simulink library "vlbi_lib"  (Simulink 7.3)
settings: Solver=ode45  SolverMode=SingleTasking  StartTime=0.0  StopTime=10.0  RelTol=1e-3
libraries: xbsIndex_r4 x437, xbsReplacements_r4 x26, simulink x3, xps_library x2
(part 1 of 2)
settings Model: Creator=rprimian  LastModifiedBy=rprimian

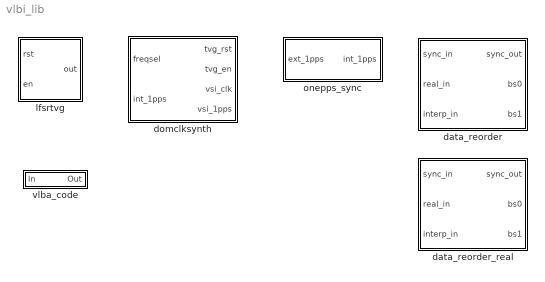
== system vlbi_lib ==
  data_reorder : Subsystem  mask{sample_width=2, vsi_clock=32 MHz}
      mask prompts: sample_width "Channel sample width:"; vsi_clock "VSI output clock rate:"
      mask init:
      | myname = gcb;
      | 
      | if (strcmp(vsi_clock, '32 MHz'))
      |     set_param([gcb, '/sync2rd'], 'latency', '4');
      |     set_param([gcb, '/rdaddrcount'], 'n_bits', '4');
      |     set_param([gcb, '/rdaddrtopslice'], 'nbits', '3');
      |     set_param([gcb, '/wraddrcount'], 'n_bits', '4');
      |     set_param([gcb, '/sync2align'], 'latency', '7');
      |     set_param([gcb, '/aligncount'], 'n_bits', '3');
      |     set_param([gcb, '/alignconst'], 'n_bits', '3');
      |     set_param([gcb, '/reorder_bram'], 'depth', '32');
      | elseif (strcmp(vsi_clock, '64 MHz'))
      |     set_param([gcb, '/sync2rd'], 'latency', '2');
      |     set_param([gcb, '/rdaddrcount'], 'n_bits', '3');
      |     set_param([gcb, '/rdaddrtopslice'], 'nbits', '2');
      |     set_param([gcb, '/wraddrcount'], 'n_bits', '3');
      |     set_param([gcb, '/sync2align'], 'latency', '5');
      |     set_param([gcb, '/aligncount'], 'n_bits', '2');
      |     set_param([gcb, '/alignconst'], 'n_bits', '2');
      |     set_param([gcb, '/reorder_bram'], 'depth', '16');
      | end
      mask StyleString: edit,popup(32 MHz|64 MHz)
  data_reorder_real : Subsystem  mask{sample_width=8, vsi_clock=32 MHz}
      mask prompts: sample_width "Channel sample width:"; vsi_clock "VSI output clock rate:"
      mask init:
      | myname = gcb;
      | 
      | if (strcmp(vsi_clock, '32 MHz'))
      |     set_param([gcb, '/restream'], 'clock_rate', '32');
      |     set_param([gcb, '/slc_wrmask'], 'bit1', '-1');
      | else
      |     set_param([gcb, '/restream'], 'clock_rate', '64');
      |     set_param([gcb, '/slc_wrmask'], 'bit1', '0');
      | end
      mask StyleString: edit,popup(32 MHz|64 MHz)
  domclksynth : Subsystem
  lfsrtvg : Subsystem
  onepps_sync : Subsystem
  vlba_code : Subsystem  mask{bitwidth=18}
      mask prompts: bitwidth "Rounding bitwidth:"
      mask Display: fprintf('z^-4')

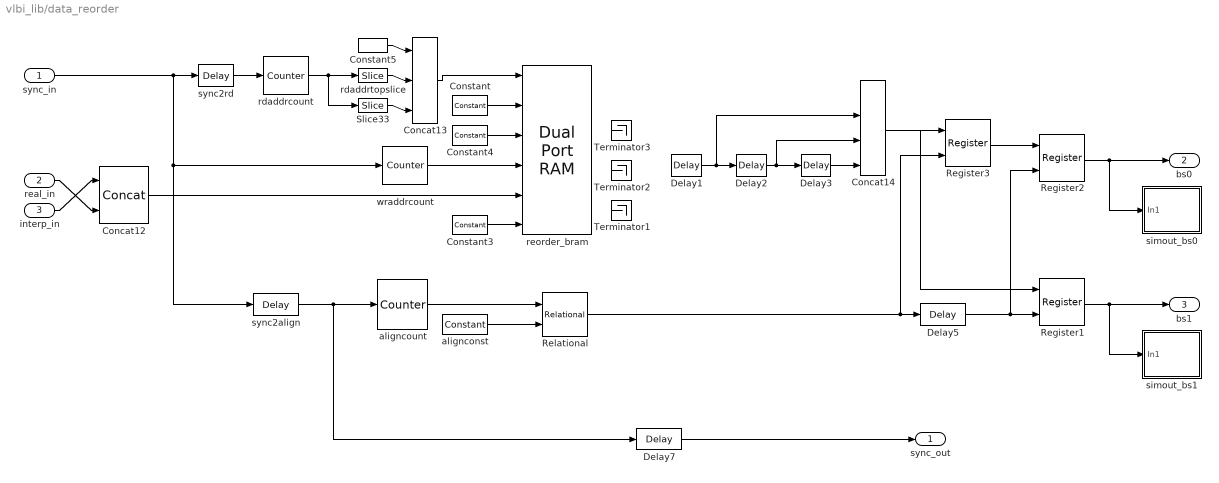
== system vlbi_lib/data_reorder ==
  sync_in : Inport  OutDataType=sfix(16)  OutScaling=2^0
  real_in : Inport  Port=2  OutDataType=sfix(16)  OutScaling=2^0
  interp_in : Inport  Port=3  OutDataType=sfix(16)  OutScaling=2^0
  Concat12 : xbsIndex_r4/Concat  num_inputs=2  dbl_ovrd=off  block_type=concat
      settings: block_version=11.3
  Concat13 : xbsIndex_r4/Concat  num_inputs=3  dbl_ovrd=off  block_type=concat
      settings: block_version=11.3
  Concat14 : xbsIndex_r4/Concat  num_inputs=4  dbl_ovrd=off  block_type=concat
      settings: block_version=11.3
  Constant : xbsIndex_r4/Constant  arith_type=Unsigned  const=0  n_bits=sample_width * 4  bin_pt=0  explicit_period=on  period=1  equ=P=C  opselect=C  inp2=PCIN>>17  opr=+  inp1=P  carry=CIN  dbl_ovrd=off  block_type=constant
      settings: block_version=11.3
  Constant3 : xbsIndex_r4/Constant  arith_type=Boolean  const=1  n_bits=1  bin_pt=0  explicit_period=on  period=1  equ=P=C  opselect=C  inp2=PCIN>>17  opr=+  inp1=P  carry=CIN  dbl_ovrd=off  block_type=constant
      settings: block_version=11.3
  Constant4 : xbsIndex_r4/Constant  arith_type=Boolean  const=0  n_bits=1024  bin_pt=0  explicit_period=on  period=1  equ=P=C  opselect=C  inp2=PCIN>>17  opr=+  inp1=P  carry=CIN  dbl_ovrd=off  block_type=constant
      settings: block_version=11.3
  Constant5 : xbsIndex_r4/Constant  arith_type=Unsigned  const=0  n_bits=1  bin_pt=0  explicit_period=on  period=1  equ=P=C  opselect=C  inp2=PCIN>>17  opr=+  inp1=P  carry=CIN  dbl_ovrd=off  block_type=constant
      settings: block_version=11.3
  Delay{1..3,7} (4 alike) : xbsIndex_r4/Delay  en=off  latency=1  dbl_ovrd=off  reg_retiming=off  block_type=delay
      settings: xl_area=[0, 0, 0, 0, 0, 0, 0]  block_version=11.3
  Delay5 : xbsIndex_r4/Delay  en=off  latency=4  dbl_ovrd=off  reg_retiming=off  block_type=delay
      settings: xl_area=[0, 0, 0, 0, 0, 0, 0]  block_version=11.3
  Register1 : xbsIndex_r4/Register  init=0  rst=off  en=on  dbl_ovrd=off  block_type=register
      settings: xl_area=[0, 0, 0, 0, 0, 0, 0]  block_version=11.3
  Register2 : xbsIndex_r4/Register  init=0  rst=off  en=on  dbl_ovrd=off  block_type=register
      settings: xl_area=[0, 0, 0, 0, 0, 0, 0]  block_version=11.3
  Register3 : xbsIndex_r4/Register  init=0  rst=off  en=on  dbl_ovrd=off  block_type=register
      settings: xl_area=[0, 0, 0, 0, 0, 0, 0]  block_version=11.3
  Relational : xbsIndex_r4/Relational  mode=a=b  en=off  latency=1  dbl_ovrd=off  block_type=relational
      settings: xl_area=[0, 0, 0, 0, 0, 0, 0]  block_version=11.3
  Slice33 : xbsIndex_r4/Slice  nbits=1  boolean_output=off  mode=Upper Bit Location + Width  bit1=0  base1=MSB of Input  bit0=0  base0=LSB of Input  dbl_ovrd=off  block_type=slice
      settings: block_version=11.3
  Terminator1 : Terminator
  Terminator2 : Terminator
  Terminator3 : Terminator
  alignconst : xbsIndex_r4/Constant  arith_type=Unsigned  const=0  n_bits=3  bin_pt=0  explicit_period=on  period=1  equ=P=C  opselect=C  inp2=PCIN>>17  opr=+  inp1=P  carry=CIN  dbl_ovrd=off  block_type=constant
      settings: block_version=11.3
  aligncount : xbsIndex_r4/Counter  cnt_type=Free Running  cnt_to=Inf  operation=Up  start_count=0  cnt_by_val=1  arith_type=Unsigned  n_bits=3  bin_pt=0  load_pin=off  rst=on  en=off  explicit_period=off  period=1  dbl_ovrd=off  use_behavioral_HDL=off  implementation=Fabric  use_rpm=on  block_type=counter
      settings: xl_area=[0, 0, 0, 0, 0, 0, 0]  block_version=11.3
  rdaddrcount : xbsIndex_r4/Counter  cnt_type=Free Running  cnt_to=Inf  operation=Up  start_count=0  cnt_by_val=1  arith_type=Unsigned  n_bits=4  bin_pt=0  load_pin=off  rst=on  en=off  explicit_period=off  period=1  dbl_ovrd=off  use_behavioral_HDL=off  implementation=Fabric  use_rpm=on  block_type=counter
      settings: xl_area=[0, 0, 0, 0, 0, 0, 0]  block_version=11.3
  rdaddrtopslice : xbsIndex_r4/Slice  nbits=3  boolean_output=off  mode=Lower Bit Location + Width  bit1=0  base1=MSB of Input  bit0=0  base0=LSB of Input  dbl_ovrd=off  block_type=slice
      settings: block_version=11.3
  reorder_bram : xbsIndex_r4/Dual Port RAM  depth=32  initVector=zeros(32)  distributed_mem=Block RAM  init_a=0  init_b=0  rst_a=off  rst_b=off  en_a=off  en_b=off  latency=1  write_mode_A=Read After Write  write_mode_B=Read After Write  dbl_ovrd=off  optimize=Area  use_rpm=off  block_type=dpram
      settings: xl_area=[0, 0, 0, 0, 0, 0, 0]  block_version=11.3
  simout_bs0 : Subsystem  mask{sample_width=sample_width}
      mask prompts: sample_width "Sample width"
  simout_bs1 : Subsystem  mask{sample_width=sample_width}
      mask prompts: sample_width "Sample width"
  sync2align : xbsIndex_r4/Delay  en=off  latency=7  dbl_ovrd=off  reg_retiming=off  block_type=delay
      settings: xl_area=[0, 0, 0, 0, 0, 0, 0]  block_version=11.3
  sync2rd : xbsIndex_r4/Delay  en=off  latency=4  dbl_ovrd=off  reg_retiming=off  block_type=delay
      settings: xl_area=[0, 0, 0, 0, 0, 0, 0]  block_version=11.3
  wraddrcount : xbsIndex_r4/Counter  cnt_type=Free Running  cnt_to=Inf  operation=Up  start_count=0  cnt_by_val=1  arith_type=Unsigned  n_bits=4  bin_pt=0  load_pin=off  rst=on  en=off  explicit_period=off  period=1  dbl_ovrd=off  use_behavioral_HDL=off  implementation=Fabric  use_rpm=on  block_type=counter
      settings: xl_area=[0, 0, 0, 0, 0, 0, 0]  block_version=11.3
  sync_out : Outport  OutDataType=sfix(16)  OutScaling=2^0
  bs0 : Outport  Port=2  OutDataType=sfix(16)  OutScaling=2^0
  bs1 : Outport  Port=3  OutDataType=sfix(16)  OutScaling=2^0
  wires:
  ? -> Terminator3/1
  Concat12/1 -> reorder_bram/5
  ? -> Terminator1/1
  Constant/1 -> reorder_bram/2
  Constant4/1 -> reorder_bram/3
  rdaddrcount/1 -> rdaddrtopslice/1, Slice33/1
  Constant5/1 -> Concat13/1
  rdaddrtopslice/1 -> Concat13/2
  Slice33/1 -> Concat13/3
  Concat13/1 -> reorder_bram/1
  wraddrcount/1 -> reorder_bram/4
  Constant3/1 -> reorder_bram/6
  Concat14/1 -> Register1/1, Register3/1
  aligncount/1 -> Relational/1
  alignconst/1 -> Relational/2
  Register2/1 -> bs0/1, simout_bs0/1(In1)
  Relational/1 -> Delay5/1, Register3/2
  Register1/1 -> bs1/1, simout_bs1/1(In1)
  Delay5/1 -> Register1/2, Register2/2
  ? -> Terminator2/1
  Register3/1 -> Register2/1
  sync_in/1 -> sync2rd/1, wraddrcount/1, sync2align/1
  sync2rd/1 -> rdaddrcount/1
  real_in/1 -> Concat12/2
  interp_in/1 -> Concat12/1
  sync2align/1 -> aligncount/1, Delay7/1
  Delay7/1 -> sync_out/1
  ? -> Delay1/1, Concat14/1
  Delay2/1 -> Delay3/1, Concat14/3
  Delay1/1 -> Delay2/1, Concat14/2
  Delay3/1 -> Concat14/4

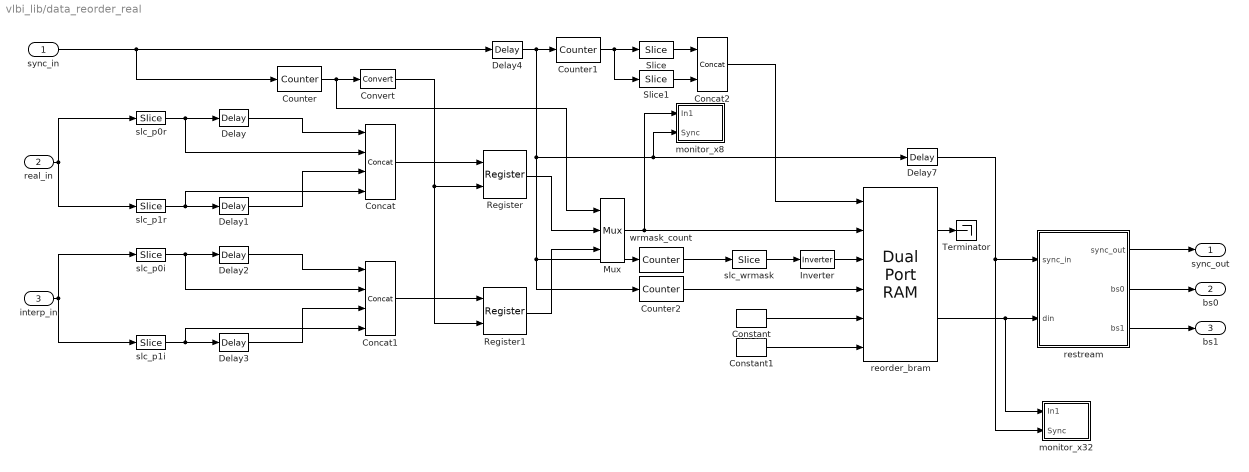
== system vlbi_lib/data_reorder_real ==
  sync_in : Inport  OutDataType=sfix(16)  OutScaling=2^0
  real_in : Inport  Port=2  OutDataType=sfix(16)  OutScaling=2^0
  interp_in : Inport  Port=3  OutDataType=sfix(16)  OutScaling=2^0
  Concat : xbsIndex_r4/Concat  num_inputs=4  dbl_ovrd=off  block_type=concat
      settings: block_version=11.3
  Concat1 : xbsIndex_r4/Concat  num_inputs=4  dbl_ovrd=off  block_type=concat
      settings: block_version=11.3
  Concat2 : xbsIndex_r4/Concat  num_inputs=2  dbl_ovrd=off  block_type=concat
      settings: block_version=11.3
  Constant : xbsIndex_r4/Constant  arith_type=Unsigned  const=0  n_bits=32*sample_width  bin_pt=0  explicit_period=on  period=1  equ=P=C  opselect=C  inp2=PCIN>>17  opr=+  inp1=P  carry=CIN  dbl_ovrd=off  block_type=constant
      settings: block_version=11.3
  Constant1 : xbsIndex_r4/Constant  arith_type=Boolean  const=0  n_bits=8*sample_width  bin_pt=0  explicit_period=on  period=1  equ=P=C  opselect=C  inp2=PCIN>>17  opr=+  inp1=P  carry=CIN  dbl_ovrd=off  block_type=constant
      settings: block_version=11.3
  Convert : xbsIndex_r4/Convert  arith_type=Boolean  n_bits=8  bin_pt=6  quantization=Truncate  overflow=Wrap  latency=0  dbl_ovrd=off  pipeline=off  block_type=convert
      settings: xl_area=[0, 0, 0, 0, 0, 0, 0]  block_version=11.3
  Counter : xbsIndex_r4/Counter  cnt_type=Free Running  cnt_to=Inf  operation=Up  start_count=0  cnt_by_val=1  arith_type=Unsigned  n_bits=1  bin_pt=0  load_pin=off  rst=on  en=off  explicit_period=off  period=1  dbl_ovrd=off  use_behavioral_HDL=off  implementation=Fabric  use_rpm=on  block_type=counter
      settings: xl_area=[0, 0, 0, 0, 0, 0, 0]  block_version=11.3
  Counter1 : xbsIndex_r4/Counter  cnt_type=Free Running  cnt_to=Inf  operation=Up  start_count=0  cnt_by_val=1  arith_type=Unsigned  n_bits=3  bin_pt=0  load_pin=off  rst=on  en=off  explicit_period=off  period=1  dbl_ovrd=off  use_behavioral_HDL=off  implementation=Fabric  use_rpm=on  block_type=counter
      settings: xl_area=[0, 0, 0, 0, 0, 0, 0]  block_version=11.3
  Counter2 : xbsIndex_r4/Counter  cnt_type=Free Running  cnt_to=Inf  operation=Up  start_count=0  cnt_by_val=1  arith_type=Unsigned  n_bits=1  bin_pt=0  load_pin=off  rst=on  en=off  explicit_period=off  period=1  dbl_ovrd=off  use_behavioral_HDL=off  implementation=Fabric  use_rpm=on  block_type=counter
      settings: xl_area=[0, 0, 0, 0, 0, 0, 0]  block_version=11.3
  Delay{,1..3} (4 alike) : xbsIndex_r4/Delay  en=off  latency=1  dbl_ovrd=off  reg_retiming=off  block_type=delay
      settings: xl_area=[0, 0, 0, 0, 0, 0, 0]  block_version=11.3
  Delay4 : xbsIndex_r4/Delay  en=off  latency=3  dbl_ovrd=off  reg_retiming=off  block_type=delay
      settings: xl_area=[0, 0, 0, 0, 0, 0, 0]  block_version=11.3
  Delay7 : xbsIndex_r4/Delay  en=off  latency=11  dbl_ovrd=off  reg_retiming=off  block_type=delay
      settings: xl_area=[0, 0, 0, 0, 0, 0, 0]  block_version=11.3
  Inverter : xbsIndex_r4/Inverter  en=off  latency=0  dbl_ovrd=off  block_type=inv
      settings: xl_area=[0, 0, 0, 0, 0, 0, 0]  block_version=11.3
  Mux : xbsIndex_r4/Mux  inputs=2  en=off  latency=1  precision=Full  arith_type="Signed  (2's comp)"  n_bits=8  bin_pt=2  quantization=Truncate  overflow=Wrap  dbl_ovrd=off  block_type=mux
      settings: xl_area=[0, 0, 0, 0, 0, 0, 0]  block_version=11.3
  Register : xbsIndex_r4/Register  init=0  rst=off  en=on  dbl_ovrd=off  block_type=register
      settings: xl_area=[0, 0, 0, 0, 0, 0, 0]  block_version=11.3
  Register1 : xbsIndex_r4/Register  init=0  rst=off  en=on  dbl_ovrd=off  block_type=register
      settings: xl_area=[0, 0, 0, 0, 0, 0, 0]  block_version=11.3
  Slice : xbsIndex_r4/Slice  nbits=1  boolean_output=off  mode=Lower Bit Location + Width  bit1=0  base1=MSB of Input  bit0=0  base0=LSB of Input  dbl_ovrd=off  block_type=slice
      settings: block_version=11.3
  Slice1 : xbsIndex_r4/Slice  nbits=2  boolean_output=off  mode=Upper Bit Location + Width  bit1=0  base1=MSB of Input  bit0=0  base0=LSB of Input  dbl_ovrd=off  block_type=slice
      settings: block_version=11.3
  Terminator : Terminator
  monitor_x32 : Subsystem
  monitor_x8 : Subsystem
  reorder_bram : xbsIndex_r4/Dual Port RAM  depth=8  initVector=zeros(2)  distributed_mem=Block RAM  init_a=0  init_b=0  rst_a=off  rst_b=off  en_a=off  en_b=off  latency=3  write_mode_A=Read Before Write  write_mode_B=Read Before Write  dbl_ovrd=off  optimize=Area  use_rpm=off  block_type=dpram
      settings: xl_area=[0, 0, 0, 0, 0, 0, 0]  block_version=11.3
  restream : Subsystem  mask{clock_rate=32}
      mask prompts: clock_rate "Clock rate (MHz)"
  slc_p0i : xbsIndex_r4/Slice  nbits=2*sample_width  boolean_output=off  mode=Upper Bit Location + Width  bit1=0  base1=MSB of Input  bit0=0  base0=LSB of Input  dbl_ovrd=off  block_type=slice
      settings: block_version=11.3
  slc_p0r : xbsIndex_r4/Slice  nbits=2*sample_width  boolean_output=off  mode=Upper Bit Location + Width  bit1=0  base1=MSB of Input  bit0=0  base0=LSB of Input  dbl_ovrd=off  block_type=slice
      settings: block_version=11.3
  slc_p1i : xbsIndex_r4/Slice  nbits=2*sample_width  boolean_output=off  mode=Upper Bit Location + Width  bit1=-2*sample_width  base1=MSB of Input  bit0=0  base0=LSB of Input  dbl_ovrd=off  block_type=slice
      settings: block_version=11.3
  slc_p1r : xbsIndex_r4/Slice  nbits=2*sample_width  boolean_output=off  mode=Upper Bit Location + Width  bit1=-2*sample_width  base1=MSB of Input  bit0=0  base0=LSB of Input  dbl_ovrd=off  block_type=slice
      settings: block_version=11.3
  slc_wrmask : xbsIndex_r4/Slice  nbits=1  boolean_output=on  mode=Upper Bit Location + Width  bit1=-1  base1=MSB of Input  bit0=0  base0=LSB of Input  dbl_ovrd=off  block_type=slice
      settings: block_version=11.3
  wrmask_count : xbsIndex_r4/Counter  cnt_type=Count Limited  cnt_to=31  operation=Up  start_count=0  cnt_by_val=1  arith_type=Unsigned  n_bits=6  bin_pt=0  load_pin=off  rst=on  en=off  explicit_period=off  period=1  dbl_ovrd=off  use_behavioral_HDL=off  implementation=Fabric  use_rpm=on  block_type=counter
      settings: xl_area=[0, 0, 0, 0, 0, 0, 0]  block_version=11.3
  sync_out : Outport  OutDataType=sfix(16)  OutScaling=2^0
  bs0 : Outport  Port=2  OutDataType=sfix(16)  OutScaling=2^0
  bs1 : Outport  Port=3  OutDataType=sfix(16)  OutScaling=2^0
  wires:
  real_in/1 -> slc_p0r/1, slc_p1r/1
  interp_in/1 -> slc_p0i/1, slc_p1i/1
  slc_p0r/1 -> Delay/1, Concat/2
  slc_p1r/1 -> Delay1/1, Concat/4
  slc_p0i/1 -> Delay2/1, Concat1/2
  slc_p1i/1 -> Delay3/1, Concat1/4
  Delay/1 -> Concat/1
  Delay1/1 -> Concat/3
  Delay2/1 -> Concat1/1
  Delay3/1 -> Concat1/3
  Concat/1 -> Register/1
  Concat1/1 -> Register1/1
  sync_in/1 -> Counter/1, Delay4/1
  Counter/1 -> Convert/1, Mux/1
  Convert/1 -> Register/2, Register1/2
  Register/1 -> Mux/2
  Register1/1 -> Mux/3
  Constant/1 -> reorder_bram/5
  Constant1/1 -> reorder_bram/6
  Mux/1 -> monitor_x8/1(In1), reorder_bram/2
  slc_wrmask/1 -> Inverter/1
  Delay4/1 -> Counter1/1, Delay7/1, monitor_x8/2(Sync), Counter2/1, wrmask_count/1
  Counter2/1 -> reorder_bram/4
  reorder_bram/1 -> Terminator/1
  Slice/1 -> Concat2/1
  Slice1/1 -> Concat2/2
  Counter1/1 -> Slice/1, Slice1/1
  Concat2/1 -> reorder_bram/1
  Delay7/1 -> restream/1(sync_in), monitor_x32/2(Sync)
  reorder_bram/2 -> restream/2(din), monitor_x32/1(In1)
  restream/1(sync_out) -> sync_out/1
  restream/2(bs0) -> bs0/1
  restream/3(bs1) -> bs1/1
  wrmask_count/1 -> slc_wrmask/1
  Inverter/1 -> reorder_bram/3

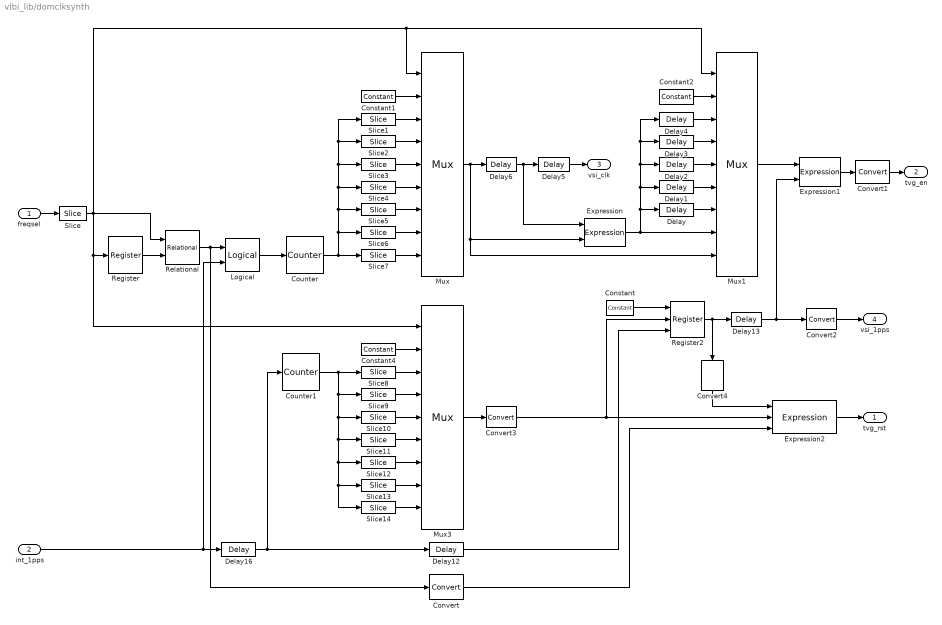
== system vlbi_lib/domclksynth ==
  freqsel : Inport  OutDataType=sfix(16)  OutScaling=2^0
  int_1pps : Inport  Port=2  OutDataType=sfix(16)  OutScaling=2^0
  Constant : xbsIndex_r4/Constant  arith_type=Unsigned  const=1  n_bits=1  bin_pt=0  explicit_period=on  period=1  equ=P=C  opselect=C  inp2=PCIN>>17  opr=+  inp1=P  carry=CIN  dbl_ovrd=off  block_type=constant
      settings: block_version=11.3
  Constant1 : xbsIndex_r4/Constant  arith_type=Unsigned  const=0  n_bits=1  bin_pt=0  explicit_period=on  period=1  equ=P=C  opselect=C  inp2=PCIN>>17  opr=+  inp1=P  carry=CIN  dbl_ovrd=off  block_type=constant
      settings: block_version=11.3
  Constant2 : xbsIndex_r4/Constant  arith_type=Unsigned  const=0  n_bits=1  bin_pt=0  explicit_period=on  period=1  equ=P=C  opselect=C  inp2=PCIN>>17  opr=+  inp1=P  carry=CIN  dbl_ovrd=off  block_type=constant
      settings: block_version=11.3
  Constant4 : xbsIndex_r4/Constant  arith_type=Unsigned  const=0  n_bits=1  bin_pt=0  explicit_period=on  period=1  equ=P=C  opselect=C  inp2=PCIN>>17  opr=+  inp1=P  carry=CIN  dbl_ovrd=off  block_type=constant
      settings: block_version=11.3
  Convert : xbsIndex_r4/Convert  arith_type=Boolean  n_bits=1  bin_pt=0  quantization=Truncate  overflow=Wrap  latency=2  dbl_ovrd=off  pipeline=off  block_type=convert
      settings: xl_area=[0, 0, 0, 0, 0, 0, 0]  block_version=11.3
  Convert{1..4} (4 alike) : xbsIndex_r4/Convert  arith_type=Boolean  n_bits=1  bin_pt=0  quantization=Truncate  overflow=Wrap  latency=0  dbl_ovrd=off  pipeline=off  block_type=convert
      settings: xl_area=[0, 0, 0, 0, 0, 0, 0]  block_version=11.3
  Counter : xbsIndex_r4/Counter  cnt_type=Free Running  cnt_to=Inf  operation=Up  start_count=0  cnt_by_val=1  arith_type=Unsigned  n_bits=8  bin_pt=0  load_pin=off  rst=on  en=off  explicit_period=on  period=1  dbl_ovrd=off  use_behavioral_HDL=off  implementation=Fabric  use_rpm=on  block_type=counter
      settings: xl_area=[0, 0, 0, 0, 0, 0, 0]  block_version=11.3
  Counter1 : xbsIndex_r4/Counter  cnt_type=Free Running  cnt_to=Inf  operation=Up  start_count=0  cnt_by_val=1  arith_type=Unsigned  n_bits=8  bin_pt=0  load_pin=off  rst=on  en=off  explicit_period=on  period=1  dbl_ovrd=off  use_behavioral_HDL=off  implementation=Fabric  use_rpm=on  block_type=counter
      settings: xl_area=[0, 0, 0, 0, 0, 0, 0]  block_version=11.3
  Delay{,5,12,16} (4 alike) : xbsIndex_r4/Delay  en=off  latency=2  dbl_ovrd=off  reg_retiming=off  block_type=delay
      settings: xl_area=[0, 0, 0, 0, 0, 0, 0]  block_version=11.3
  Delay1 : xbsIndex_r4/Delay  en=off  latency=6  dbl_ovrd=off  reg_retiming=off  block_type=delay
      settings: xl_area=[0, 0, 0, 0, 0, 0, 0]  block_version=11.3
  Delay13 : xbsIndex_r4/Delay  en=off  latency=1  dbl_ovrd=off  reg_retiming=off  block_type=delay
      settings: xl_area=[0, 0, 0, 0, 0, 0, 0]  block_version=11.3
  Delay2 : xbsIndex_r4/Delay  en=off  latency=14  dbl_ovrd=off  reg_retiming=off  block_type=delay
      settings: xl_area=[0, 0, 0, 0, 0, 0, 0]  block_version=11.3
  Delay3 : xbsIndex_r4/Delay  en=off  latency=30  dbl_ovrd=off  reg_retiming=off  block_type=delay
      settings: xl_area=[0, 0, 0, 0, 0, 0, 0]  block_version=11.3
  Delay4 : xbsIndex_r4/Delay  en=off  latency=62  dbl_ovrd=off  reg_retiming=off  block_type=delay
      settings: xl_area=[0, 0, 0, 0, 0, 0, 0]  block_version=11.3
  Delay6 : xbsIndex_r4/Delay  en=off  latency=1  dbl_ovrd=off  reg_retiming=off  block_type=delay
      settings: xl_area=[0, 0, 0, 0, 0, 0, 0]  block_version=11.3
  Expression : xbsIndex_r4/Expression  expression=~a & b  align_bp=on  en=off  latency=1  precision=Full  arith_type=Unsigned  n_bits=8  bin_pt=2  dbl_ovrd=off  block_type=expr
      settings: xl_area=[0, 0, 0, 0, 0, 0, 0]  block_version=11.3
  Expression1 : xbsIndex_r4/Expression  expression=a & ~b  align_bp=on  en=off  latency=1  precision=Full  arith_type=Unsigned  n_bits=8  bin_pt=2  dbl_ovrd=off  block_type=expr
      settings: xl_area=[0, 0, 0, 0, 0, 0, 0]  block_version=11.3
  Expression2 : xbsIndex_r4/Expression  expression=(a & b) | c  align_bp=on  en=off  latency=1  precision=Full  arith_type=Unsigned  n_bits=8  bin_pt=2  dbl_ovrd=off  block_type=expr
      settings: xl_area=[0, 0, 0, 0, 0, 0, 0]  block_version=11.3
  Logical : xbsIndex_r4/Logical  logical_function=OR  inputs=2  en=off  latency=1  precision=Full  arith_type=Unsigned  n_bits=8  bin_pt=2  align_bp=on  dbl_ovrd=off  block_type=logical
      settings: xl_area=[0, 0, 0, 0, 0, 0, 0]  block_version=11.3
  Mux : xbsIndex_r4/Mux  inputs=8  en=off  latency=1  precision=Full  arith_type="Signed  (2's comp)"  n_bits=8  bin_pt=2  quantization=Truncate  overflow=Wrap  dbl_ovrd=off  block_type=mux
      settings: xl_area=[0, 0, 0, 0, 0, 0, 0]  block_version=11.3
  Mux1 : xbsIndex_r4/Mux  inputs=8  en=off  latency=1  precision=Full  arith_type="Signed  (2's comp)"  n_bits=8  bin_pt=2  quantization=Truncate  overflow=Wrap  dbl_ovrd=off  block_type=mux
      settings: xl_area=[0, 0, 0, 0, 0, 0, 0]  block_version=11.3
  Mux3 : xbsIndex_r4/Mux  inputs=8  en=off  latency=1  precision=Full  arith_type="Signed  (2's comp)"  n_bits=8  bin_pt=2  quantization=Truncate  overflow=Wrap  dbl_ovrd=off  block_type=mux
      settings: xl_area=[0, 0, 0, 0, 0, 0, 0]  block_version=11.3
  Register : xbsIndex_r4/Register  init=0  rst=off  en=off  dbl_ovrd=off  block_type=register
      settings: xl_area=[0, 0, 0, 0, 0, 0, 0]  block_version=11.3
  Register2 : xbsIndex_r4/Register  init=0  rst=on  en=on  dbl_ovrd=off  block_type=register
      settings: xl_area=[0, 0, 0, 0, 0, 0, 0]  block_version=11.3
  Relational : xbsIndex_r4/Relational  mode=a!=b  en=off  latency=1  dbl_ovrd=off  block_type=relational
      settings: xl_area=[0, 0, 0, 0, 0, 0, 0]  block_version=11.3
  Slice : xbsIndex_r4/Slice  nbits=3  boolean_output=off  mode=Lower Bit Location + Width  bit1=0  base1=MSB of Input  bit0=0  base0=LSB of Input  dbl_ovrd=off  block_type=slice
      settings: block_version=11.3
  Slice1 : xbsIndex_r4/Slice  nbits=1  boolean_output=off  mode=Upper Bit Location + Width  bit1=-1  base1=MSB of Input  bit0=0  base0=LSB of Input  dbl_ovrd=off  block_type=slice
      settings: block_version=11.3
  Slice10 : xbsIndex_r4/Slice  nbits=1  boolean_output=off  mode=Upper Bit Location + Width  bit1=-2  base1=MSB of Input  bit0=0  base0=LSB of Input  dbl_ovrd=off  block_type=slice
      settings: block_version=11.3
  Slice11 : xbsIndex_r4/Slice  nbits=1  boolean_output=off  mode=Upper Bit Location + Width  bit1=-3  base1=MSB of Input  bit0=0  base0=LSB of Input  dbl_ovrd=off  block_type=slice
      settings: block_version=11.3
  Slice12 : xbsIndex_r4/Slice  nbits=1  boolean_output=off  mode=Upper Bit Location + Width  bit1=-4  base1=MSB of Input  bit0=0  base0=LSB of Input  dbl_ovrd=off  block_type=slice
      settings: block_version=11.3
  Slice13 : xbsIndex_r4/Slice  nbits=1  boolean_output=off  mode=Upper Bit Location + Width  bit1=-5  base1=MSB of Input  bit0=0  base0=LSB of Input  dbl_ovrd=off  block_type=slice
      settings: block_version=11.3
  Slice14 : xbsIndex_r4/Slice  nbits=1  boolean_output=off  mode=Upper Bit Location + Width  bit1=-6  base1=MSB of Input  bit0=0  base0=LSB of Input  dbl_ovrd=off  block_type=slice
      settings: block_version=11.3
  Slice2 : xbsIndex_r4/Slice  nbits=1  boolean_output=off  mode=Upper Bit Location + Width  bit1=-2  base1=MSB of Input  bit0=0  base0=LSB of Input  dbl_ovrd=off  block_type=slice
      settings: block_version=11.3
  Slice3 : xbsIndex_r4/Slice  nbits=1  boolean_output=off  mode=Upper Bit Location + Width  bit1=-3  base1=MSB of Input  bit0=0  base0=LSB of Input  dbl_ovrd=off  block_type=slice
      settings: block_version=11.3
  Slice4 : xbsIndex_r4/Slice  nbits=1  boolean_output=off  mode=Upper Bit Location + Width  bit1=-4  base1=MSB of Input  bit0=0  base0=LSB of Input  dbl_ovrd=off  block_type=slice
      settings: block_version=11.3
  Slice5 : xbsIndex_r4/Slice  nbits=1  boolean_output=off  mode=Upper Bit Location + Width  bit1=-5  base1=MSB of Input  bit0=0  base0=LSB of Input  dbl_ovrd=off  block_type=slice
      settings: block_version=11.3
  Slice6 : xbsIndex_r4/Slice  nbits=1  boolean_output=off  mode=Upper Bit Location + Width  bit1=-6  base1=MSB of Input  bit0=0  base0=LSB of Input  dbl_ovrd=off  block_type=slice
      settings: block_version=11.3
  Slice7 : xbsIndex_r4/Slice  nbits=1  boolean_output=off  mode=Upper Bit Location + Width  bit1=-7  base1=MSB of Input  bit0=0  base0=LSB of Input  dbl_ovrd=off  block_type=slice
      settings: block_version=11.3
  Slice8 : xbsIndex_r4/Slice  nbits=1  boolean_output=off  mode=Upper Bit Location + Width  bit1=0  base1=MSB of Input  bit0=0  base0=LSB of Input  dbl_ovrd=off  block_type=slice
      settings: block_version=11.3
  Slice9 : xbsIndex_r4/Slice  nbits=1  boolean_output=off  mode=Upper Bit Location + Width  bit1=-1  base1=MSB of Input  bit0=0  base0=LSB of Input  dbl_ovrd=off  block_type=slice
      settings: block_version=11.3
  tvg_rst : Outport  OutDataType=sfix(16)  OutScaling=2^0
  tvg_en : Outport  Port=2  OutDataType=sfix(16)  OutScaling=2^0
  vsi_clk : Outport  Port=3  OutDataType=sfix(16)  OutScaling=2^0
  vsi_1pps : Outport  Port=4  OutDataType=sfix(16)  OutScaling=2^0
  wires:
  Delay16/1 -> Counter1/1, Delay12/1
  Counter1/1 -> Slice14/1, Slice13/1, Slice12/1, Slice11/1, Slice10/1, Slice9/1, Slice8/1
  Convert3/1 -> Register2/2, Expression2/2
  Mux3/1 -> Convert3/1
  Slice14/1 -> Mux3/9
  Slice13/1 -> Mux3/8
  Slice12/1 -> Mux3/7
  Slice11/1 -> Mux3/6
  Slice10/1 -> Mux3/5
  Slice9/1 -> Mux3/4
  Slice8/1 -> Mux3/3
  Constant4/1 -> Mux3/2
  Delay12/1 -> Register2/3
  Delay5/1 -> vsi_clk/1
  Slice/1 -> Mux3/1, Register/1, Mux1/1, Mux/1, Relational/1
  Counter/1 -> Slice6/1, Slice4/1, Slice3/1, Slice2/1, Slice1/1, Slice5/1, Slice7/1
  Delay6/1 -> Delay5/1, Expression/1
  Delay13/1 -> Expression1/2, Convert2/1
  Expression1/1 -> Convert1/1
  Mux1/1 -> Expression1/1
  Relational/1 -> Convert/1, Logical/1
  Logical/1 -> Counter/1
  Mux/1 -> Mux1/9, Expression/2, Delay6/1
  Slice7/1 -> Mux/9
  Slice6/1 -> Mux/8
  Slice5/1 -> Mux/7
  Slice4/1 -> Mux/6
  Slice3/1 -> Mux/5
  Slice2/1 -> Mux/4
  Slice1/1 -> Mux/3
  Constant1/1 -> Mux/2
  Register/1 -> Relational/2
  freqsel/1 -> Slice/1
  Expression/1 -> Mux1/8, Delay4/1, Delay3/1, Delay2/1, Delay1/1, Delay/1
  Constant2/1 -> Mux1/2
  Delay4/1 -> Mux1/3
  Delay3/1 -> Mux1/4
  Delay2/1 -> Mux1/5
  Delay1/1 -> Mux1/6
  Delay/1 -> Mux1/7
  Convert1/1 -> tvg_en/1
  Register2/1 -> Delay13/1, Convert4/1
  Constant/1 -> Register2/1
  Convert2/1 -> vsi_1pps/1
  int_1pps/1 -> Delay16/1, Logical/2
  Expression2/1 -> tvg_rst/1
  Convert/1 -> Expression2/3
  Convert4/1 -> Expression2/1

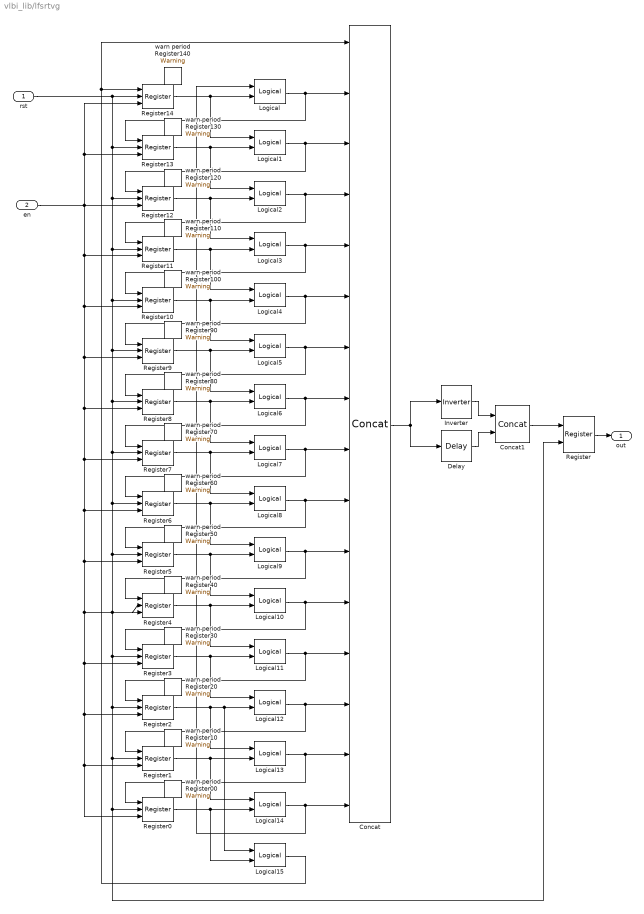
== system vlbi_lib/lfsrtvg ==
  rst : Inport  OutDataType=sfix(16)  OutScaling=2^0
  en : Inport  Port=2  OutDataType=sfix(16)  OutScaling=2^0
  Concat : xbsIndex_r4/Concat  num_inputs=16  dbl_ovrd=off  block_type=concat
      settings: block_version=11.3
  Concat1 : xbsIndex_r4/Concat  num_inputs=2  dbl_ovrd=off  block_type=concat
      settings: block_version=11.3
  Delay : xbsIndex_r4/Delay  en=off  latency=0  dbl_ovrd=off  reg_retiming=off  block_type=delay
      settings: xl_area=[0, 0, 0, 0, 0, 0, 0]  block_version=11.3
  Inverter : xbsIndex_r4/Inverter  en=off  latency=0  dbl_ovrd=off  block_type=inv
      settings: xl_area=[0, 0, 0, 0, 0, 0, 0]  block_version=11.3
  Logical{,1..15} (16 alike) : xbsIndex_r4/Logical  logical_function=XOR  inputs=2  en=off  latency=0  precision=Full  arith_type=Unsigned  n_bits=8  bin_pt=2  align_bp=on  dbl_ovrd=off  block_type=logical
      settings: xl_area=[0, 0, 0, 0, 0, 0, 0]  block_version=11.3
  Register : xbsIndex_r4/Register  init=3221176320  rst=on  en=off  dbl_ovrd=off  block_type=register
      settings: xl_area=[0, 0, 0, 0, 0, 0, 0]  block_version=11.3
  Register{0..14} (15 alike) : xbsIndex_r4/Register  init=1  rst=on  en=on  dbl_ovrd=off  block_type=register
      settings: xl_area=[0, 0, 0, 0, 0, 0, 0]  block_version=11.3
  warn period Register00 : xbsReplacements_r4/Warning  SystemSampleTime=-1  period=1
  warn period Register{10,20,30,40,50,60,70,80,90,100,110,120,130,140} (14 alike) : xbsReplacements_r4/Warning  SystemSampleTime=-1  period=1
  out : Outport  OutDataType=sfix(16)  OutScaling=2^0
  wires:
  Register/1 -> out/1
  Concat1/1 -> Register/1
  Delay/1 -> Concat1/2
  Inverter/1 -> Concat1/1
  Concat/1 -> Delay/1, Inverter/1
  Logical13/1 -> Concat/15, Register0/1
  Logical12/1 -> Concat/14, Register1/1
  Logical11/1 -> Concat/13, Register2/1
  Logical10/1 -> Concat/12, Register3/1
  Logical9/1 -> Concat/11, Register4/1
  Logical8/1 -> Concat/10, Register5/1
  Logical7/1 -> Concat/9, Register6/1
  Logical6/1 -> Concat/8, Register7/1
  Logical5/1 -> Concat/7, Register8/1
  Logical4/1 -> Concat/6, Register9/1
  Logical3/1 -> Concat/5, Register10/1
  Logical2/1 -> Concat/4, Register11/1
  Logical1/1 -> Concat/3, Register12/1
  Logical/1 -> Concat/2, Register13/1
  Logical15/1 -> Concat/1, Register14/1
  Logical14/1 -> Concat/16, Logical/1
  Register0/1 -> Logical15/2, Logical14/2
  Register1/1 -> Logical13/2, Logical14/1
  Register2/1 -> Logical15/1, Logical12/2, Logical13/1
  Register3/1 -> Logical11/2, Logical12/1
  Register4/1 -> Logical10/2, Logical11/1
  Register5/1 -> Logical9/2, Logical10/1
  Register6/1 -> Logical8/2, Logical9/1
  Register7/1 -> Logical7/2, Logical8/1
  Register8/1 -> Logical6/2, Logical7/1
  Register9/1 -> Logical5/2, Logical6/1
  Register10/1 -> Logical4/2, Logical5/1
  Register11/1 -> Logical3/2, Logical4/1
  Register12/1 -> Logical2/2, Logical3/1
  Register13/1 -> Logical1/2, Logical2/1
  Register14/1 -> Logical/2, Logical1/1
  rst/1 -> Register14/2, Register/2, Register0/2, Register1/2, Register2/2, Register3/2, Register4/2, Register5/2, Register6/2, Register7/2, Register8/2, Register9/2, Register10/2, Register11/2, Register12/2, Register13/2
  en/1 -> Register14/3, Register13/3, Register12/3, Register11/3, Register10/3, Register7/3, Register6/3, Register5/3, Register4/3, Register3/3, Register2/3, Register1/3, Register0/3, Register8/3, Register9/3

== system vlbi_lib/onepps_sync ==
  ext_1pps : Inport  OutDataType=sfix(16)  OutScaling=2^0
  Step : Step  Time=200  Before=1  After=0  SampleTime=1
  Terminator : Terminator
  arm1pps : xps_library/software register  Tag=xps:sw_reg  SystemSampleTime=-1  io_dir=From Processor  arith_type=Unsigned  bitwidth=32  bin_pt=0  sample_period=1  gw_name=vlbi_lib_onepps_sync_arm1pps_user_data_out
  arm1pps_ack : xps_library/software register  Tag=xps:sw_reg  SystemSampleTime=-1  io_dir=To Processor  arith_type=Unsigned  bitwidth=32  bin_pt=0  sample_period=1  gw_name=vlbi_lib_onepps_sync_arm1pps_ack_user_data_in
  armshake : Subsystem
  int_1pps_gen : Subsystem
  int_1pps : Outport  OutDataType=sfix(16)  OutScaling=2^0
  wires:
  arm1pps_ack/1 -> Terminator/1
  armshake/2(arm_ack) -> arm1pps_ack/1
  armshake/1(rst_1pps) -> int_1pps_gen/1(rst)
  Step/1 -> arm1pps/1
  arm1pps/1 -> armshake/2(ext_arm1pps)
  ext_1pps/1 -> armshake/1(ext_1pps)
  int_1pps_gen/1(1pps) -> int_1pps/1

== system vlbi_lib/vlba_code ==
  In : Inport  OutDataType=sfix(16)  OutScaling=2^0
  Concat : xbsIndex_r4/Concat  num_inputs=2  dbl_ovrd=off  block_type=concat
      settings: block_version=11.3
  Constant : xbsIndex_r4/Constant  arith_type=Signed (2's comp)  const=0  n_bits=bitwidth  bin_pt=bitwidth-1  explicit_period=on  period=1  equ=P=C  opselect=C  inp2=PCIN>>17  opr=+  inp1=P  carry=CIN  dbl_ovrd=off  block_type=constant
      settings: block_version=11.3
  Constant1 : xbsIndex_r4/Constant  arith_type=Signed (2's comp)  const=-.5  n_bits=bitwidth  bin_pt=bitwidth-1  explicit_period=on  period=1  equ=P=C  opselect=C  inp2=PCIN>>17  opr=+  inp1=P  carry=CIN  dbl_ovrd=off  block_type=constant
      settings: block_version=11.3
  Constant2 : xbsIndex_r4/Constant  arith_type=Signed (2's comp)  const=.5  n_bits=bitwidth  bin_pt=bitwidth-1  explicit_period=on  period=1  equ=P=C  opselect=C  inp2=PCIN>>17  opr=+  inp1=P  carry=CIN  dbl_ovrd=off  block_type=constant
      settings: block_version=11.3
  Convert1 : xbsIndex_r4/Convert  arith_type="Signed  (2's comp)"  n_bits=bitwidth  bin_pt=bitwidth-1  quantization=Truncate  overflow=Saturate  latency=2  dbl_ovrd=off  pipeline=on  block_type=convert
      settings: xl_area=[0, 0, 0, 0, 0, 0, 0]  block_version=11.3
  Delay : xbsIndex_r4/Delay  en=off  latency=1  dbl_ovrd=off  reg_retiming=off  block_type=delay
      settings: xl_area=[0, 0, 0, 0, 0, 0, 0]  block_version=11.3
  Mux : xbsIndex_r4/Mux  inputs=2  en=off  latency=1  precision=Full  arith_type="Signed  (2's comp)"  n_bits=8  bin_pt=2  quantization=Truncate  overflow=Wrap  dbl_ovrd=off  block_type=mux
      settings: xl_area=[0, 0, 0, 0, 0, 0, 0]  block_version=11.3
  Relational : xbsIndex_r4/Relational  mode=a>=b  en=off  latency=3  dbl_ovrd=off  block_type=relational
      settings: xl_area=[0, 0, 0, 0, 0, 0, 0]  block_version=11.3
  Relational1 : xbsIndex_r4/Relational  mode=a>=b  en=off  latency=3  dbl_ovrd=off  block_type=relational
      settings: xl_area=[0, 0, 0, 0, 0, 0, 0]  block_version=11.3
  Relational2 : xbsIndex_r4/Relational  mode=a>=b  en=off  latency=3  dbl_ovrd=off  block_type=relational
      settings: xl_area=[0, 0, 0, 0, 0, 0, 0]  block_version=11.3
  Out : Outport  OutDataType=sfix(16)  OutScaling=2^0
  wires:
  Delay/1 -> Concat/2
  Relational2/1 -> Mux/3
  Relational1/1 -> Mux/2
  Relational/1 -> Delay/1, Mux/1
  Mux/1 -> Concat/1
  Constant2/1 -> Relational2/2
  Constant1/1 -> Relational1/2
  Constant/1 -> Relational/2
  Convert1/1 -> Relational2/1, Relational1/1, Relational/1
  Concat/1 -> Out/1
  In/1 -> Convert1/1

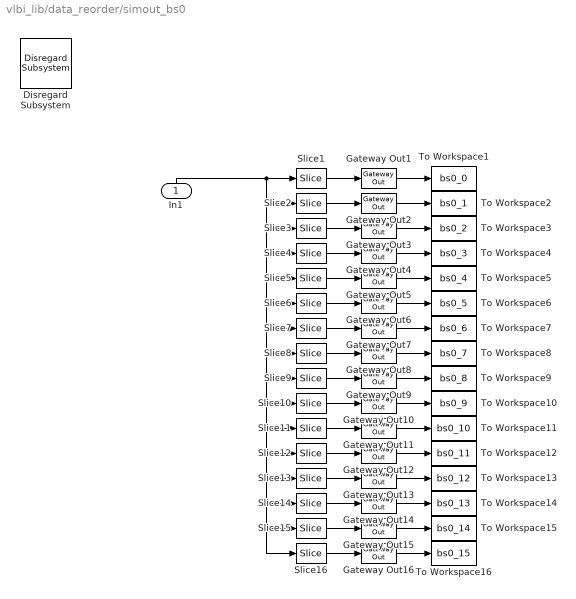
== system vlbi_lib/data_reorder/simout_bs0 ==
  In1 : Inport  OutDataType=sfix(16)  OutScaling=2^0
  Disregard Subsystem : xbsIndex_r4/Disregard Subsystem  Tag=discardX  block_type=disregard
      settings: block_version=11.3
  Gateway Out{1..16} (16 alike) : xbsIndex_r4/Gateway Out  hdl_port=off  timing_constraint=None  locs_specified=off  LOCs={}  block_type=gatewayout
      settings: infoedit="Gateway out block.  Converts Xilinx fixed point inputs into ouputs of type Simulink integer, double, or fixed point.<br><br>Hardware notes:  In hardware these blocks become top level output ports or are discarded, depending on how they are configured."  xl_area=[0, 0, 0, 0, 0, 0, 0]  block_version=11.3
  Slice1 : xbsIndex_r4/Slice  nbits=sample_width  boolean_output=off  mode=Upper Bit Location + Width  bit1=sample_width * 0  base1=MSB of Input  bit0=0  base0=LSB of Input  dbl_ovrd=off  block_type=slice
      settings: block_version=11.3
  Slice10 : xbsIndex_r4/Slice  nbits=sample_width  boolean_output=off  mode=Upper Bit Location + Width  bit1=sample_width * -9  base1=MSB of Input  bit0=0  base0=LSB of Input  dbl_ovrd=off  block_type=slice
      settings: block_version=11.3
  Slice11 : xbsIndex_r4/Slice  nbits=sample_width  boolean_output=off  mode=Upper Bit Location + Width  bit1=sample_width * -10  base1=MSB of Input  bit0=0  base0=LSB of Input  dbl_ovrd=off  block_type=slice
      settings: block_version=11.3
  Slice12 : xbsIndex_r4/Slice  nbits=sample_width  boolean_output=off  mode=Upper Bit Location + Width  bit1=sample_width * -11  base1=MSB of Input  bit0=0  base0=LSB of Input  dbl_ovrd=off  block_type=slice
      settings: block_version=11.3
  Slice13 : xbsIndex_r4/Slice  nbits=sample_width  boolean_output=off  mode=Upper Bit Location + Width  bit1=sample_width * -12  base1=MSB of Input  bit0=0  base0=LSB of Input  dbl_ovrd=off  block_type=slice
      settings: block_version=11.3
  Slice14 : xbsIndex_r4/Slice  nbits=sample_width  boolean_output=off  mode=Upper Bit Location + Width  bit1=sample_width * -13  base1=MSB of Input  bit0=0  base0=LSB of Input  dbl_ovrd=off  block_type=slice
      settings: block_version=11.3
  Slice15 : xbsIndex_r4/Slice  nbits=sample_width  boolean_output=off  mode=Upper Bit Location + Width  bit1=sample_width * -14  base1=MSB of Input  bit0=0  base0=LSB of Input  dbl_ovrd=off  block_type=slice
      settings: block_version=11.3
  Slice16 : xbsIndex_r4/Slice  nbits=sample_width  boolean_output=off  mode=Upper Bit Location + Width  bit1=sample_width * -15  base1=MSB of Input  bit0=0  base0=LSB of Input  dbl_ovrd=off  block_type=slice
      settings: block_version=11.3
  Slice2 : xbsIndex_r4/Slice  nbits=sample_width  boolean_output=off  mode=Upper Bit Location + Width  bit1=sample_width * -1  base1=MSB of Input  bit0=0  base0=LSB of Input  dbl_ovrd=off  block_type=slice
      settings: block_version=11.3
  Slice3 : xbsIndex_r4/Slice  nbits=sample_width  boolean_output=off  mode=Upper Bit Location + Width  bit1=sample_width * -2  base1=MSB of Input  bit0=0  base0=LSB of Input  dbl_ovrd=off  block_type=slice
      settings: block_version=11.3
  Slice4 : xbsIndex_r4/Slice  nbits=sample_width  boolean_output=off  mode=Upper Bit Location + Width  bit1=sample_width * -3  base1=MSB of Input  bit0=0  base0=LSB of Input  dbl_ovrd=off  block_type=slice
      settings: block_version=11.3
  Slice5 : xbsIndex_r4/Slice  nbits=sample_width  boolean_output=off  mode=Upper Bit Location + Width  bit1=sample_width * -4  base1=MSB of Input  bit0=0  base0=LSB of Input  dbl_ovrd=off  block_type=slice
      settings: block_version=11.3
  Slice6 : xbsIndex_r4/Slice  nbits=sample_width  boolean_output=off  mode=Upper Bit Location + Width  bit1=sample_width * -5  base1=MSB of Input  bit0=0  base0=LSB of Input  dbl_ovrd=off  block_type=slice
      settings: block_version=11.3
  Slice7 : xbsIndex_r4/Slice  nbits=sample_width  boolean_output=off  mode=Upper Bit Location + Width  bit1=sample_width * -6  base1=MSB of Input  bit0=0  base0=LSB of Input  dbl_ovrd=off  block_type=slice
      settings: block_version=11.3
  Slice8 : xbsIndex_r4/Slice  nbits=sample_width  boolean_output=off  mode=Upper Bit Location + Width  bit1=sample_width * -7  base1=MSB of Input  bit0=0  base0=LSB of Input  dbl_ovrd=off  block_type=slice
      settings: block_version=11.3
  Slice9 : xbsIndex_r4/Slice  nbits=sample_width  boolean_output=off  mode=Upper Bit Location + Width  bit1=sample_width * -8  base1=MSB of Input  bit0=0  base0=LSB of Input  dbl_ovrd=off  block_type=slice
      settings: block_version=11.3
  To Workspace1 : ToWorkspace  VariableName=bs0_0  SampleTime=-1  SaveFormat=Array
  To Workspace10 : ToWorkspace  VariableName=bs0_9  SampleTime=-1  SaveFormat=Array
  To Workspace11 : ToWorkspace  VariableName=bs0_10  SampleTime=-1  SaveFormat=Array
  To Workspace12 : ToWorkspace  VariableName=bs0_11  SampleTime=-1  SaveFormat=Array
  To Workspace13 : ToWorkspace  VariableName=bs0_12  SampleTime=-1  SaveFormat=Array
  To Workspace14 : ToWorkspace  VariableName=bs0_13  SampleTime=-1  SaveFormat=Array
  To Workspace15 : ToWorkspace  VariableName=bs0_14  SampleTime=-1  SaveFormat=Array
  To Workspace16 : ToWorkspace  VariableName=bs0_15  SampleTime=-1  SaveFormat=Array
  To Workspace2 : ToWorkspace  VariableName=bs0_1  SampleTime=-1  SaveFormat=Array
  To Workspace3 : ToWorkspace  VariableName=bs0_2  SampleTime=-1  SaveFormat=Array
  To Workspace4 : ToWorkspace  VariableName=bs0_3  SampleTime=-1  SaveFormat=Array
  To Workspace5 : ToWorkspace  VariableName=bs0_4  SampleTime=-1  SaveFormat=Array
  To Workspace6 : ToWorkspace  VariableName=bs0_5  SampleTime=-1  SaveFormat=Array
  To Workspace7 : ToWorkspace  VariableName=bs0_6  SampleTime=-1  SaveFormat=Array
  To Workspace8 : ToWorkspace  VariableName=bs0_7  SampleTime=-1  SaveFormat=Array
  To Workspace9 : ToWorkspace  VariableName=bs0_8  SampleTime=-1  SaveFormat=Array
  wires:
  Slice1/1 -> Gateway Out1/1
  Slice2/1 -> Gateway Out2/1
  Slice3/1 -> Gateway Out3/1
  Slice4/1 -> Gateway Out4/1
  Slice5/1 -> Gateway Out5/1
  Slice6/1 -> Gateway Out6/1
  Slice7/1 -> Gateway Out7/1
  Gateway Out1/1 -> To Workspace1/1
  Gateway Out2/1 -> To Workspace2/1
  Gateway Out3/1 -> To Workspace3/1
  Gateway Out4/1 -> To Workspace4/1
  Gateway Out5/1 -> To Workspace5/1
  Gateway Out6/1 -> To Workspace6/1
  Gateway Out7/1 -> To Workspace7/1
  Slice8/1 -> Gateway Out8/1
  Gateway Out8/1 -> To Workspace8/1
  Slice9/1 -> Gateway Out9/1
  Gateway Out9/1 -> To Workspace9/1
  Slice10/1 -> Gateway Out10/1
  Gateway Out10/1 -> To Workspace10/1
  Slice11/1 -> Gateway Out11/1
  Gateway Out11/1 -> To Workspace11/1
  Slice12/1 -> Gateway Out12/1
  Gateway Out12/1 -> To Workspace12/1
  Slice13/1 -> Gateway Out13/1
  Gateway Out13/1 -> To Workspace13/1
  Slice14/1 -> Gateway Out14/1
  Gateway Out14/1 -> To Workspace14/1
  Slice15/1 -> Gateway Out15/1
  Gateway Out15/1 -> To Workspace15/1
  Slice16/1 -> Gateway Out16/1
  Gateway Out16/1 -> To Workspace16/1
  In1/1 -> Slice2/1, Slice3/1, Slice4/1, Slice5/1, Slice6/1, Slice7/1, Slice8/1, Slice9/1, Slice10/1, Slice11/1, Slice12/1, Slice13/1, Slice14/1, Slice15/1, Slice16/1, Slice1/1

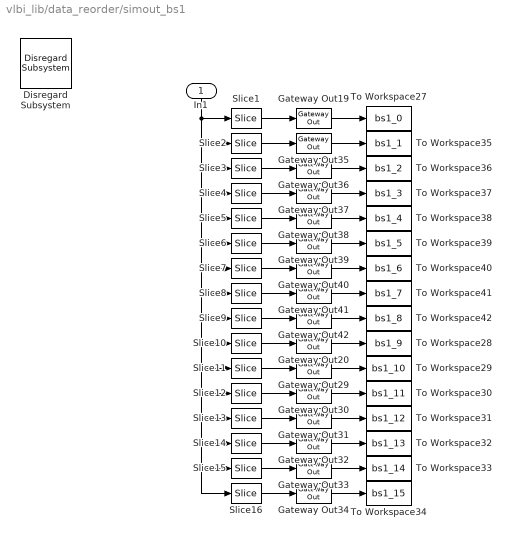
== system vlbi_lib/data_reorder/simout_bs1 ==
  In1 : Inport  OutDataType=sfix(16)  OutScaling=2^0
  Disregard Subsystem : xbsIndex_r4/Disregard Subsystem  Tag=discardX  block_type=disregard
      settings: block_version=11.3
  Gateway Out{19..20,29..42} (16 alike) : xbsIndex_r4/Gateway Out  hdl_port=off  timing_constraint=None  locs_specified=off  LOCs={}  block_type=gatewayout
      settings: infoedit="Gateway out block.  Converts Xilinx fixed point inputs into ouputs of type Simulink integer, double, or fixed point.<br><br>Hardware notes:  In hardware these blocks become top level output ports or are discarded, depending on how they are configured."  xl_area=[0, 0, 0, 0, 0, 0, 0]  block_version=11.3
  Slice1 : xbsIndex_r4/Slice  nbits=sample_width  boolean_output=off  mode=Upper Bit Location + Width  bit1=sample_width * 0  base1=MSB of Input  bit0=0  base0=LSB of Input  dbl_ovrd=off  block_type=slice
      settings: block_version=11.3
  Slice10 : xbsIndex_r4/Slice  nbits=sample_width  boolean_output=off  mode=Upper Bit Location + Width  bit1=sample_width * -9  base1=MSB of Input  bit0=0  base0=LSB of Input  dbl_ovrd=off  block_type=slice
      settings: block_version=11.3
  Slice11 : xbsIndex_r4/Slice  nbits=sample_width  boolean_output=off  mode=Upper Bit Location + Width  bit1=sample_width * -10  base1=MSB of Input  bit0=0  base0=LSB of Input  dbl_ovrd=off  block_type=slice
      settings: block_version=11.3
  Slice12 : xbsIndex_r4/Slice  nbits=sample_width  boolean_output=off  mode=Upper Bit Location + Width  bit1=sample_width * -11  base1=MSB of Input  bit0=0  base0=LSB of Input  dbl_ovrd=off  block_type=slice
      settings: block_version=11.3
  Slice13 : xbsIndex_r4/Slice  nbits=sample_width  boolean_output=off  mode=Upper Bit Location + Width  bit1=sample_width * -12  base1=MSB of Input  bit0=0  base0=LSB of Input  dbl_ovrd=off  block_type=slice
      settings: block_version=11.3
  Slice14 : xbsIndex_r4/Slice  nbits=sample_width  boolean_output=off  mode=Upper Bit Location + Width  bit1=sample_width * -13  base1=MSB of Input  bit0=0  base0=LSB of Input  dbl_ovrd=off  block_type=slice
      settings: block_version=11.3
  Slice15 : xbsIndex_r4/Slice  nbits=sample_width  boolean_output=off  mode=Upper Bit Location + Width  bit1=sample_width * -14  base1=MSB of Input  bit0=0  base0=LSB of Input  dbl_ovrd=off  block_type=slice
      settings: block_version=11.3
  Slice16 : xbsIndex_r4/Slice  nbits=sample_width  boolean_output=off  mode=Upper Bit Location + Width  bit1=sample_width * -15  base1=MSB of Input  bit0=0  base0=LSB of Input  dbl_ovrd=off  block_type=slice
      settings: block_version=11.3
  Slice2 : xbsIndex_r4/Slice  nbits=sample_width  boolean_output=off  mode=Upper Bit Location + Width  bit1=sample_width * -1  base1=MSB of Input  bit0=0  base0=LSB of Input  dbl_ovrd=off  block_type=slice
      settings: block_version=11.3
  Slice3 : xbsIndex_r4/Slice  nbits=sample_width  boolean_output=off  mode=Upper Bit Location + Width  bit1=sample_width * -2  base1=MSB of Input  bit0=0  base0=LSB of Input  dbl_ovrd=off  block_type=slice
      settings: block_version=11.3
  Slice4 : xbsIndex_r4/Slice  nbits=sample_width  boolean_output=off  mode=Upper Bit Location + Width  bit1=sample_width * -3  base1=MSB of Input  bit0=0  base0=LSB of Input  dbl_ovrd=off  block_type=slice
      settings: block_version=11.3
  Slice5 : xbsIndex_r4/Slice  nbits=sample_width  boolean_output=off  mode=Upper Bit Location + Width  bit1=sample_width * -4  base1=MSB of Input  bit0=0  base0=LSB of Input  dbl_ovrd=off  block_type=slice
      settings: block_version=11.3
  Slice6 : xbsIndex_r4/Slice  nbits=sample_width  boolean_output=off  mode=Upper Bit Location + Width  bit1=sample_width * -5  base1=MSB of Input  bit0=0  base0=LSB of Input  dbl_ovrd=off  block_type=slice
      settings: block_version=11.3
  Slice7 : xbsIndex_r4/Slice  nbits=sample_width  boolean_output=off  mode=Upper Bit Location + Width  bit1=sample_width * -6  base1=MSB of Input  bit0=0  base0=LSB of Input  dbl_ovrd=off  block_type=slice
      settings: block_version=11.3
  Slice8 : xbsIndex_r4/Slice  nbits=sample_width  boolean_output=off  mode=Upper Bit Location + Width  bit1=sample_width * -7  base1=MSB of Input  bit0=0  base0=LSB of Input  dbl_ovrd=off  block_type=slice
      settings: block_version=11.3
  Slice9 : xbsIndex_r4/Slice  nbits=sample_width  boolean_output=off  mode=Upper Bit Location + Width  bit1=sample_width * -8  base1=MSB of Input  bit0=0  base0=LSB of Input  dbl_ovrd=off  block_type=slice
      settings: block_version=11.3
  To Workspace27 : ToWorkspace  VariableName=bs1_0  SampleTime=-1  SaveFormat=Array
  To Workspace28 : ToWorkspace  VariableName=bs1_9  SampleTime=-1  SaveFormat=Array
  To Workspace29 : ToWorkspace  VariableName=bs1_10  SampleTime=-1  SaveFormat=Array
  To Workspace30 : ToWorkspace  VariableName=bs1_11  SampleTime=-1  SaveFormat=Array
  To Workspace31 : ToWorkspace  VariableName=bs1_12  SampleTime=-1  SaveFormat=Array
  To Workspace32 : ToWorkspace  VariableName=bs1_13  SampleTime=-1  SaveFormat=Array
  To Workspace33 : ToWorkspace  VariableName=bs1_14  SampleTime=-1  SaveFormat=Array
  To Workspace34 : ToWorkspace  VariableName=bs1_15  SampleTime=-1  SaveFormat=Array
  To Workspace35 : ToWorkspace  VariableName=bs1_1  SampleTime=-1  SaveFormat=Array
  To Workspace36 : ToWorkspace  VariableName=bs1_2  SampleTime=-1  SaveFormat=Array
  To Workspace37 : ToWorkspace  VariableName=bs1_3  SampleTime=-1  SaveFormat=Array
  To Workspace38 : ToWorkspace  VariableName=bs1_4  SampleTime=-1  SaveFormat=Array
  To Workspace39 : ToWorkspace  VariableName=bs1_5  SampleTime=-1  SaveFormat=Array
  To Workspace40 : ToWorkspace  VariableName=bs1_6  SampleTime=-1  SaveFormat=Array
  To Workspace41 : ToWorkspace  VariableName=bs1_7  SampleTime=-1  SaveFormat=Array
  To Workspace42 : ToWorkspace  VariableName=bs1_8  SampleTime=-1  SaveFormat=Array
  wires:
  Slice1/1 -> Gateway Out19/1
  Slice2/1 -> Gateway Out35/1
  Slice3/1 -> Gateway Out36/1
  Slice4/1 -> Gateway Out37/1
  Slice5/1 -> Gateway Out38/1
  Slice6/1 -> Gateway Out39/1
  Slice7/1 -> Gateway Out40/1
  Gateway Out19/1 -> To Workspace27/1
  Gateway Out35/1 -> To Workspace35/1
  Gateway Out36/1 -> To Workspace36/1
  Gateway Out37/1 -> To Workspace37/1
  Gateway Out38/1 -> To Workspace38/1
  Gateway Out39/1 -> To Workspace39/1
  Gateway Out40/1 -> To Workspace40/1
  Slice8/1 -> Gateway Out41/1
  Gateway Out41/1 -> To Workspace41/1
  Slice9/1 -> Gateway Out42/1
  Gateway Out42/1 -> To Workspace42/1
  Slice10/1 -> Gateway Out20/1
  Gateway Out20/1 -> To Workspace28/1
  Slice11/1 -> Gateway Out29/1
  Gateway Out29/1 -> To Workspace29/1
  Slice12/1 -> Gateway Out30/1
  Gateway Out30/1 -> To Workspace30/1
  Slice13/1 -> Gateway Out31/1
  Gateway Out31/1 -> To Workspace31/1
  Slice14/1 -> Gateway Out32/1
  Gateway Out32/1 -> To Workspace32/1
  Slice15/1 -> Gateway Out33/1
  Gateway Out33/1 -> To Workspace33/1
  Slice16/1 -> Gateway Out34/1
  Gateway Out34/1 -> To Workspace34/1
  In1/1 -> Slice15/1, Slice16/1, Slice14/1, Slice13/1, Slice12/1, Slice11/1, Slice10/1, Slice9/1, Slice8/1, Slice7/1, Slice6/1, Slice5/1, Slice4/1, Slice3/1, Slice2/1, Slice1/1
